simulink model "s1"  (R2015a)
settings: Solver=ode45  StartTime=0.02  StopTime=100.0  FixedStep=0  RelTol=1e-3
libraries: simulink x2, discretizing x2
settings Model: Creator=Dorota  LastModifiedBy=Dorota
settings SFSimCC: SimBuildMode=sf_make_clean
settings SFSimCC: SimCustomHeaderCode=|
  | #include "./PID.h"
  | #include "./test.h"
settings SFSimCC: SimCustomInitializer=|
  | //PID_init(1, 0.012, 0.12, 0, 0.2, 0);
  | init_test();
settings SFSimCC: SimUserSources=|
  | ./PID.c
  | ./test.c

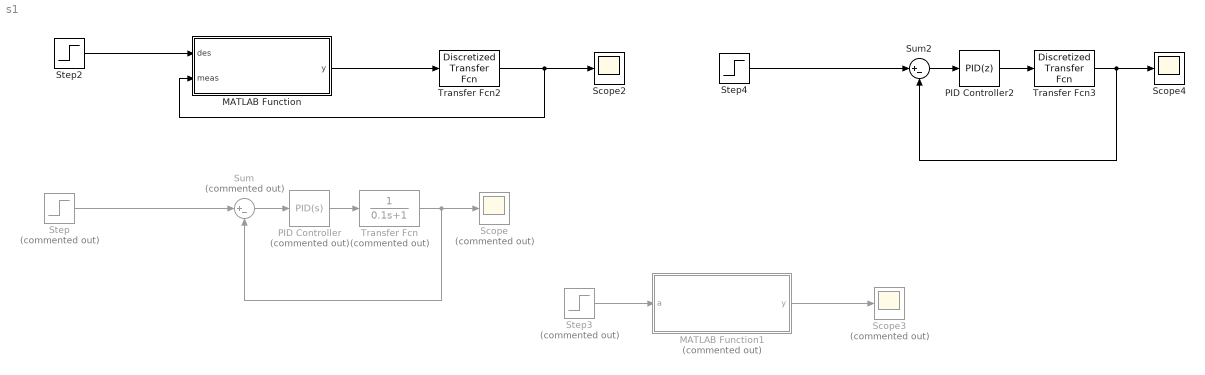
== system s1 ==
  MATLAB Function : MATLAB Function  TreatAsAtomicUnit=on
  MATLAB Function1 : MATLAB Function  Commented=on  TreatAsAtomicUnit=on
  PID Controller : simulink/Continuous/PID Controller  Commented=on  Controller=PID  TimeDomain=Continuous-time  SampleTime=-1  IntegratorMethod=Forward Euler  FilterMethod=Forward Euler  Form=Parallel  UseFilter=on  ControllerParametersSource=internal  P=1.3375803137951  I=26.7355246643925  D=-0.00485758916096801  N=37.8094165182863  InitialConditionSource=internal  InitialConditionForIntegrator=0  InitialConditionForFilter=0  ExternalReset=none  LimitOutput=off  UpperSaturationLimit=inf  LowerSaturationLimit=-inf  LinearizeAsGain=on  AntiWindupMode=none  Kb=1  TrackingMode=off  Kt=1  PParamMin=[]  PParamMax=[]  IParamMin=[]  IParamMax=[]  DParamMin=[]  DParamMax=[]  NParamMin=[]  NParamMax=[]  KbParamMin=[]  KbParamMax=[]  KtParamMin=[]  KtParamMax=[]  POutMin=[]  POutMax=[]  IOutMin=[]  IOutMax=[]  DOutMin=[]  DOutMax=[]  NOutMin=[]  NOutMax=[]  KbOutMin=[]  KbOutMax=[]  KtOutMin=[]  KtOutMax=[]  IntegratorOutMin=[]  IntegratorOutMax=[]  FilterOutMin=[]  FilterOutMax=[]  SumOutMin=[]  SumOutMax=[]  SumI1OutMin=[]  SumI1OutMax=[]  SumI2OutMin=[]  SumI2OutMax=[]  SumI3OutMin=[]  SumI3OutMax=[]  SumDOutMin=[]  SumDOutMax=[]  SaturationOutMin=[]  SaturationOutMax=[]  IntegratorContinuousStateAttributes=''  IntegratorStateMustResolveToSignalObject=off  IntegratorRTWStateStorageClass=Auto  FilterContinuousStateAttributes=''  FilterStateMustResolveToSignalObject=off  FilterRTWStateStorageClass=Auto  DifferentiatorICPrevScaledInput=0  DifferentiatorOutMin=[]  DifferentiatorOutMax=[]
  PID Controller2 : simulink/Continuous/PID Controller  Controller=PID  TimeDomain=Discrete-time  SampleTime=0.020000000000000001  IntegratorMethod=Forward Euler  FilterMethod=Forward Euler  Form=Parallel  UseFilter=on  ControllerParametersSource=internal  P=0.012  I=0.12  D=0  N=100  InitialConditionSource=internal  InitialConditionForIntegrator=0  InitialConditionForFilter=0  ExternalReset=none  LimitOutput=off  UpperSaturationLimit=inf  LowerSaturationLimit=-inf  LinearizeAsGain=on  AntiWindupMode=none  Kb=1  TrackingMode=off  Kt=1  PParamMin=[]  PParamMax=[]  IParamMin=[]  IParamMax=[]  DParamMin=[]  DParamMax=[]  NParamMin=[]  NParamMax=[]  KbParamMin=[]  KbParamMax=[]  KtParamMin=[]  KtParamMax=[]  POutMin=[]  POutMax=[]  IOutMin=[]  IOutMax=[]  DOutMin=[]  DOutMax=[]  NOutMin=[]  NOutMax=[]  KbOutMin=[]  KbOutMax=[]  KtOutMin=[]  KtOutMax=[]  IntegratorOutMin=[]  IntegratorOutMax=[]  FilterOutMin=[]  FilterOutMax=[]  SumOutMin=[]  SumOutMax=[]  SumI1OutMin=[]  SumI1OutMax=[]  SumI2OutMin=[]  SumI2OutMax=[]  SumI3OutMin=[]  SumI3OutMax=[]  SumDOutMin=[]  SumDOutMax=[]  SaturationOutMin=[]  SaturationOutMax=[]  IntegratorContinuousStateAttributes=''  IntegratorStateMustResolveToSignalObject=off  IntegratorRTWStateStorageClass=Auto  FilterContinuousStateAttributes=''  FilterStateMustResolveToSignalObject=off  FilterRTWStateStorageClass=Auto  DifferentiatorICPrevScaledInput=0  DifferentiatorOutMin=[]  DifferentiatorOutMax=[]
  Scope : Scope  Commented=on
  Scope2 : Scope
      settings: SaveName=ScopeData2
  Scope3 : Scope  Commented=on
      settings: TimeRange=99.80000000000001  YMin=-1  YMax=1  SaveName=ScopeData3
  Scope4 : Scope
      settings: SaveName=ScopeData4
  Step : Step  Commented=on  SampleTime=0
  Step2 : Step  SampleTime=0.02  mask(DiscretizedSource){}
      mask init:
      | %zoh
  Step3 : Step  Commented=on  SampleTime=0.2  mask(DiscretizedSource){}
      mask init:
      | %zoh
  Step4 : Step  SampleTime=0.02  mask(DiscretizedSource){}
      mask init:
      | %zoh
  Sum : Sum  Commented=on  Inputs=|+-
  Sum2 : Sum  Inputs=|+-
  Transfer Fcn : TransferFcn  Commented=on  Denominator=[0.1 1]
  Transfer Fcn2 : discretizing/Discretized Transfer Fcn  Numerator=[1]  Denominator=[1 0.1 1]  AbsTol=auto  SampleTime=0.02  method=zoh  Wc=1
  Transfer Fcn3 : discretizing/Discretized Transfer Fcn  Numerator=[1]  Denominator=[1 0.1 1]  AbsTol=auto  SampleTime=0.2  method=zoh  Wc=1
  wires:
  Transfer Fcn/1 -> Sum/2, Scope/1
  Step/1 -> Sum/1
  PID Controller/1 -> Transfer Fcn/1
  Sum/1 -> PID Controller/1
  Step2/1 -> MATLAB Function/1(des)
  MATLAB Function/1(y) -> Transfer Fcn2/1
  Transfer Fcn2/1 -> MATLAB Function/2(meas), Scope2/1
  Step3/1 -> MATLAB Function1/1(a)
  MATLAB Function1/1(y) -> Scope3/1
  Transfer Fcn3/1 -> Sum2/2, Scope4/1
  Step4/1 -> Sum2/1
  PID Controller2/1 -> Transfer Fcn3/1
  Sum2/1 -> PID Controller2/1

== matlab function s1/MATLAB Function1 ==
  data: y output; a input

function y = test(a)
    y = double(0);
    y = coder.ceval('test_test', a);
end

== matlab function s1/MATLAB Function ==
  data: y output; des input; meas input

function y = test (des, meas)
    y = double(0);
    y = coder.ceval('test', 2, single(des), single(meas));
end
